simulink library "TestLibrary"  (R2017a)
settings: Solver=VariableStepAuto  StartTime=0.0  StopTime=10.0  RelTol=1e-3
settings Model: Creator=ptracton  LastModifiedBy=ptracton

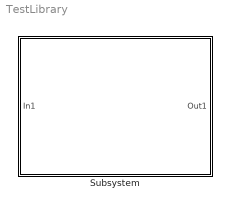
== system TestLibrary ==
  Subsystem : Subsystem

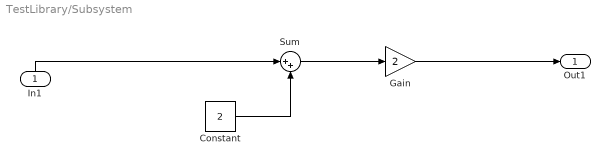
== system TestLibrary/Subsystem ==
  In1 : Inport
  Constant : Constant  Value=2
  Gain : Gain  Gain=2
  Sum : Sum  Inputs=|++
  Out1 : Outport
  wires:
  Gain/1 -> Out1/1
  Constant/1 -> Sum/2
  Sum/1 -> Gain/1
  In1/1 -> Sum/1
